simulink model "PTB_BatteryElectricVehicles"  (R2018b)
settings: Solver=ode23tb  StartTime=0.0  StopTime=3158  FixedStep=.001  RelTol=1e-5
model workspace (MAT data in the model file):
  Cd = 0.3
  DrCycles.C505 = [0 1 2 3 4 5 6 7 8 9 10 11 ... (1012 elements, 506x2)]
  DrCycles.FTP = [0 1 2 3 4 5 6 7 8 9 10 11 ... (4956 elements, 2478x2)]
  DrCycles.UDDS = [0 1 2 3 4 5 6 7 8 9 10 11 ... (2746 elements, 1373x2)]
  DrCycles.HWFET = [0 1 2 3 4 5 6 7 8 9 10 11 ... (1532 elements, 766x2)]
  DrCycles.US06 = [0 1 2 3 4 5 6 7 8 9 10 11 ... (1194 elements, 597x2)]
  DrCycles.US06City = [0 1 2 3 4 5 6 7 8 9 10 11 ... (466 elements, 233x2)]
  DrCycles.US06Hwy = [0 1 2 3 4 5 6 7 8 9 10 11 ... (742 elements, 371x2)]
  DriveCycleTime = 3158
  Drive_Cycle = Simulink.LookupTable
  Drive_Cycle.Table = Simulink.lookuptable.Table
  Drive_Cycle.Table.Value = [0 5 10 10 15 15 15 15 20 20 20 20 ... (3158 elements, 3158x1)]
  Drive_Cycle.Table.Dimensions = [3158 1]
  Drive_Cycle.Table.DataType = 'double'
  Drive_Cycle.Table.FieldName = 'Speed'
  Drive_Cycle.Breakpoints = Simulink.lookuptable.Breakpoint
  Drive_Cycle.Breakpoints.Value = [1 2 3 4 5 6 7 8 9 10 11 12 ... (3158 elements, 1x3158)]
  Drive_Cycle.Breakpoints.TunableSizeName = 'N1'
  Drive_Cycle.Breakpoints.Dimensions = [1 3158]
  Drive_Cycle.Breakpoints.DataType = 'double'
  Drive_Cycle.Breakpoints.FieldName = 'Time'
  Drive_Cycle.SupportTunableSize = 0
  Drive_Cycle.StructTypeInfo = Simulink.lookuptable.StructTypeInfo
  Drive_Cycle.StructTypeInfo.Name = 'Drive_Cycle'
  Drive_Cycle.StructTypeInfo.DataScope = 'Auto'
  I = 1
  Kbr = 5000
  P = 200
  axle_b = 10
  axle_k = 0.3
  bevAxle_wc = 400
  bevNp = 1
  bevNs = 8
  diffRatio = 1
  diffRatio1 = 1
  motorMaxTorqueNm = [0.6; 0.6; 0.8; 0.9; 2.2; 2.9; 5.1; 7.8; 11.3; 15.3; 20; 25; 35.4; 41.2; 47.2; 53.4; 66.2; 71.6; 77.2; 82.2; 87.8; 93.1; 98.3; 104; 109.4; 114.6; 120.1; 125.4; 131.1; 137.1; 144.2; 150.1; 155.4; 162.5; 168.1; 173.4; 178.2; 184.5; 190.6; 190.6]
  motorSpeedRadPs = [90.118; 90.118; 90.118; 90.118; 90.01333333; 89.804; 89.49; 89.07133333; 88.65266667; 88.12933333; 87.39666667; 86.87333333; 86.24533333; 85.722; 85.094; 84.25666667; 63.21866667; 57.462; 53.17066667; 49.612; 45.63466667; 41.97133333; 38.72666667; 35.90066667; 33.284; 30.772; 28.36466667; 26.062; 23.96866667; 21.77066667; 19.25866667; 17.47933333; 15.59533333; 13.816; 11.932; 10.25733333; 8.478; 6.594; 4.396]
  vehicleMass = 365
  wheelRadius = 0.3
undefined symbols (not defined in the file): Driver, Wheels_Driver_VehDyn_Lib
libraries: autolibshared x3, simulink x2, autolibdatasheetbattery x1, autolibmappedmotor x1
(part 1 of 3)
settings Model: PauseTimes=2  ParameterArgumentNames=motorMaxTorqueNm  OrderedModelArguments=off  Creator=ogden.michael  LastModifiedBy=ahmed
settings SolverCC: AlgebraicLoopSolver=LineSearch
settings DebuggingCC: AlgebraicLoopMsg=none  LibraryContextMissingDiagnostic=none
settings SFSimCC: SimUseLocalCustomCode=off
settings RTWCC: RTWUseLocalCustomCode=off
settings CodeAppCC: StateflowObjectComments=on
settings SimscapeCC: SimscapeNormalizeSystem=off

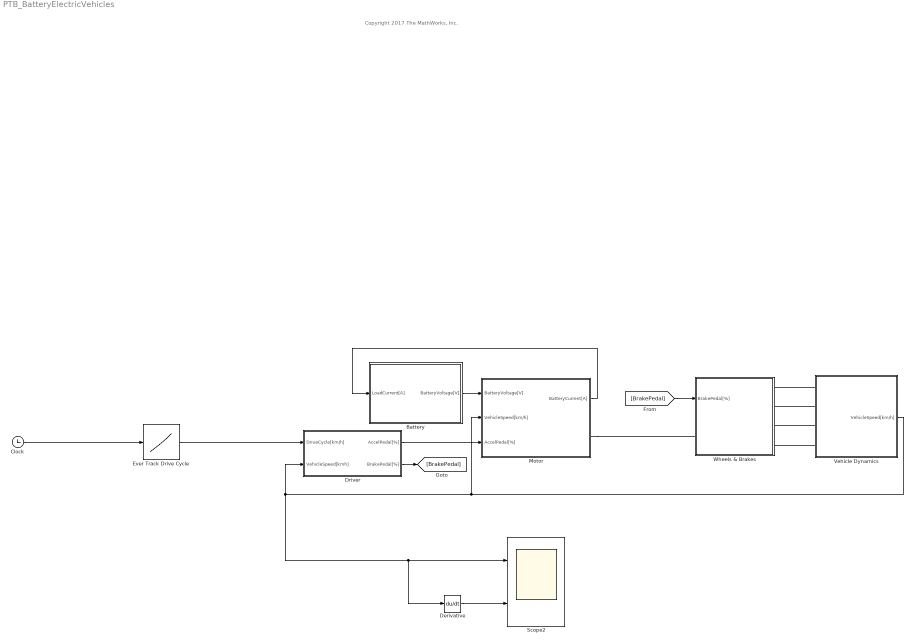
== system PTB_BatteryElectricVehicles ==
  note: Copyright 2017 The MathWorks, Inc.
  Battery : Subsystem
  Clock : Clock
  Derivative : Derivative
  "Driver " : Subsystem  AncestorBlock=Wheels_Driver_VehDyn_Lib/Driver
  Ever Track Drive Cycle : Lookup_n-D  NumberOfTableDimensions=1  DataSpecification=Lookup table object  LookupTableObject=Drive_Cycle  BreakpointsForDimension1=[-5:5]  Table=tanh([-5:5])  InternalRulePriority=Speed  RndMeth=Simplest  InputSameDT=on
  Motor : Subsystem
  Scope2 : Scope  NumInputPorts=2
  Vehicle Dynamics : Subsystem  AncestorBlock=Wheels_Driver_VehDyn_Lib/Vehicle Dynamics
  "Wheels & Brakes " : Subsystem  AncestorBlock=Wheels_Driver_VehDyn_Lib/Wheels & Brakes
  wires:
  [BrakePedal] -> "Wheels & Brakes "/1(BrakePedal[%])
  Battery/1(BatteryVoltage[V]) -> Motor/1(BatteryVoltage[V])
  "Driver "/1(AccelPedal[%]) -> Motor/3(AccelPedal[%])
  "Driver "/2(BrakePedal[%]) -> [BrakePedal]
  Motor/1(BatteryCurrent[A]) -> Battery/1(LoadCurrent[A])
  Clock/1 -> Ever Track Drive Cycle/1
  Vehicle Dynamics/1(VehicleSpeed[km/h]) -> Derivative/1, Scope2/1, "Driver "/2(VehicleSpeed[kmh]), Motor/2(VehicleSpeed[km/h])
  Ever Track Drive Cycle/1 -> "Driver "/1(" DriveCycle[km/h]")
  Derivative/1 -> Scope2/2
  connections:
  Motor/RConn1 -- "Wheels & Brakes "/LConn1
  Vehicle Dynamics/LConn3 -- "Wheels & Brakes "/RConn3
  Vehicle Dynamics/LConn1 -- "Wheels & Brakes "/RConn1
  Vehicle Dynamics/LConn4 -- "Wheels & Brakes "/RConn4
  Vehicle Dynamics/LConn2 -- "Wheels & Brakes "/RConn2

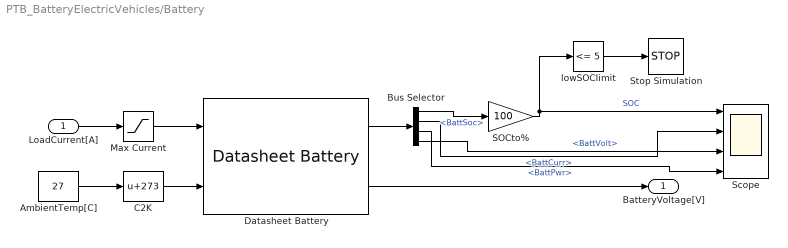
== system PTB_BatteryElectricVehicles/Battery ==
  LoadCurrent[A] : Inport
  AmbientTemp[C] : Constant  Value=27
  Bus Selector : BusSelector  OutputSignals=BattSoc,BattCurr,BattPwr,BattVolt
  C2K : Bias  Bias=273
  Datasheet Battery : autolibdatasheetbattery/Datasheet Battery  CapacityCtrl=Parameter  OutputVlt=Unfiltered  BattChargeMax=80  Em=|  CapLUTBp=|  RInt="[ 0.002789  0.002789;0.002789 0.002789]"  BattTempBp=[300 305]  CapSOCBp=[0 1]  Ns=bevNs  Np=bevNp  BattCapInit=80  Tc=1/1000  Vinit=4.221
      Em=|
      | [5.92
      | 6.22
      | 6.44
      | 6.46
      | 6.54
      | 6.56
      | 6.6
      | 6.6
      | 6.6
      | 6.6
      | 6.6
      | 6.6
      | 6.6
      | 6.6
      | 6.6
      | 6.66
      | 6.66
      | 6.66
      | 6.66
      | 6.7
      | 6.84
      | ]
      CapLUTBp=|
      | [0
      | 0.05
      | 0.1
      | 0.15
      | 0.2
      | 0.25
      | 0.3
      | 0.35
      | 0.4
      | 0.45
      | 0.5
      | 0.55
      | 0.6
      | 0.65
      | 0.7
      | 0.75
      | 0.8
      | 0.85
      | 0.9
      | 0.95
      | 1
      | ]
      settings: SourceProductName=Powertrain Blockset  SourceProductBaseCode=PW
  Max Current : Saturate  UpperLimit=180  LowerLimit=0
  SOCto% : Gain  Gain=100
  Scope : Scope  NumInputPorts=4
  Stop Simulation : Stop
  lowSOClimit : simulink/Logic and Bit Operations/Compare To Constant  relop=<=  const=5  OutDataTypeStr=boolean
  BatteryVoltage[V] : Outport
  wires:
  Datasheet Battery/1 -> Bus Selector/1
  AmbientTemp[C]/1 -> C2K/1
  Datasheet Battery/2 -> BatteryVoltage[V]/1
  C2K/1 -> Datasheet Battery/2
  SOCto%/1 -> lowSOClimit/1, Scope/1  "SOC"
  Bus Selector/1 -> SOCto%/1  "<BattSoc>"
  LoadCurrent[A]/1 -> Max Current/1
  lowSOClimit/1 -> Stop Simulation/1
  Bus Selector/2 -> Scope/2  "<BattCurr>"
  Bus Selector/3 -> Scope/4  "<BattPwr>"
  Bus Selector/4 -> Scope/3  "<BattVolt>"
  Max Current/1 -> Datasheet Battery/1

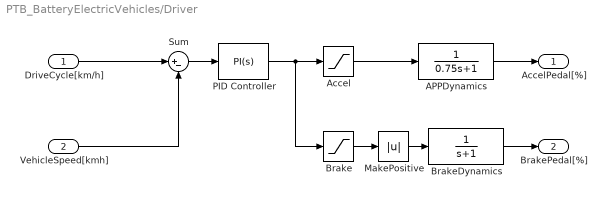
== system PTB_BatteryElectricVehicles/Driver  ==
  " DriveCycle[km/h]" : Inport
  VehicleSpeed[kmh] : Inport  Port=2
  APPDynamics : TransferFcn  Denominator=[0.75 1]
  Accel : Saturate  UpperLimit=100  LowerLimit=0
  Brake : Saturate  UpperLimit=0  LowerLimit=-100
  BrakeDynamics : TransferFcn  Denominator=[1 1]
  MakePositive : Abs
  PID Controller : simulink/Continuous/PID Controller  Controller=PI  Form=Parallel  TimeDomain=Continuous-time  SampleTime=-1  IntegratorMethod=Forward Euler  FilterMethod=Forward Euler  ControllerParametersSource=internal  P=P  I=I  D=0  UseFilter=on  N=100  TunerSelectOption=Transfer Function Based (PID Tuner App)  InitialConditionSource=internal  InitialConditionForIntegrator=0  InitialConditionForFilter=0  DifferentiatorICPrevScaledInput=0  ExternalReset=none  TrackingMode=off  Kt=1  LimitOutput=on  UpperSaturationLimit=100  LowerSaturationLimit=-100  LinearizeAsGain=on  AntiWindupMode=none  Kb=1  POutMin=[]  POutMax=[]  IOutMin=[]  IOutMax=[]  DOutMin=[]  DOutMax=[]  NOutMin=[]  NOutMax=[]  SumOutMin=[]  SumOutMax=[]  SaturationOutMin=[]  SaturationOutMax=[]  PParamMin=[]  PParamMax=[]  IParamMin=[]  IParamMax=[]  DParamMin=[]  DParamMax=[]  NParamMin=[]  NParamMax=[]  KbParamMin=[]  KbParamMax=[]  KtParamMin=[]  KtParamMax=[]  KbOutMin=[]  KbOutMax=[]  KtOutMin=[]  KtOutMax=[]  IntegratorOutMin=[]  IntegratorOutMax=[]  FilterOutMin=[]  FilterOutMax=[]  SumI1OutMin=[]  SumI1OutMax=[]  SumI2OutMin=[]  SumI2OutMax=[]  SumI3OutMin=[]  SumI3OutMax=[]  SumI4OutMin=[]  SumI4OutMax=[]  SumDOutMin=[]  SumDOutMax=[]  DifferentiatorOutMin=[]  DifferentiatorOutMax=[]  FilterDiffOutCoefMin=[]  FilterDiffOutCoefMax=[]  ReciprocalOutMin=[]  ReciprocalOutMax=[]  SumDenOutMin=[]  SumDenOutMax=[]  SumNumOutMin=[]  SumNumOutMax=[]  DivideOutMin=[]  DivideOutMax=[]  IntegratorContinuousStateAttributes=''  IntegratorStateMustResolveToSignalObject=off  IntegratorRTWStateStorageClass=Auto  FilterContinuousStateAttributes=''  FilterStateMustResolveToSignalObject=off  FilterRTWStateStorageClass=Auto  ParallelPVariant=InternalParameters  IdealPVariant=Disabled  IVariant=InternalParameters  DVariant=Disabled  IntegratorVariant=Continuous  SatVariant=Enabled  AWVariant=Passthrough  PCopyVariant=Disabled  TRVariant=Disabled  FdbkBlocksVariant=Forward  IdealPFdbkVariant=Disabled  SatFdbkVariant=Disabled  DerivativeFilterVariant=Disabled  NVariant=Disabled  NCopyVariant=Disabled_SignalSpec  FilterICVariant=Disabled  IntegratorICVariant=InternalICs  ExternalResetVariant=Disabled  TRSumVariant=Passthrough  SumFdbkVariant=Disabled  SumVariant=Sum_PI
  Sum : Sum  Inputs=|+-
  AccelPedal[%] : Outport
  BrakePedal[%] : Outport  Port=2
  wires:
  " DriveCycle[km/h]"/1 -> Sum/1
  VehicleSpeed[kmh]/1 -> Sum/2
  PID Controller/1 -> Accel/1, Brake/1
  Sum/1 -> PID Controller/1
  Brake/1 -> MakePositive/1
  Accel/1 -> APPDynamics/1
  MakePositive/1 -> BrakeDynamics/1
  APPDynamics/1 -> AccelPedal[%]/1
  BrakeDynamics/1 -> BrakePedal[%]/1

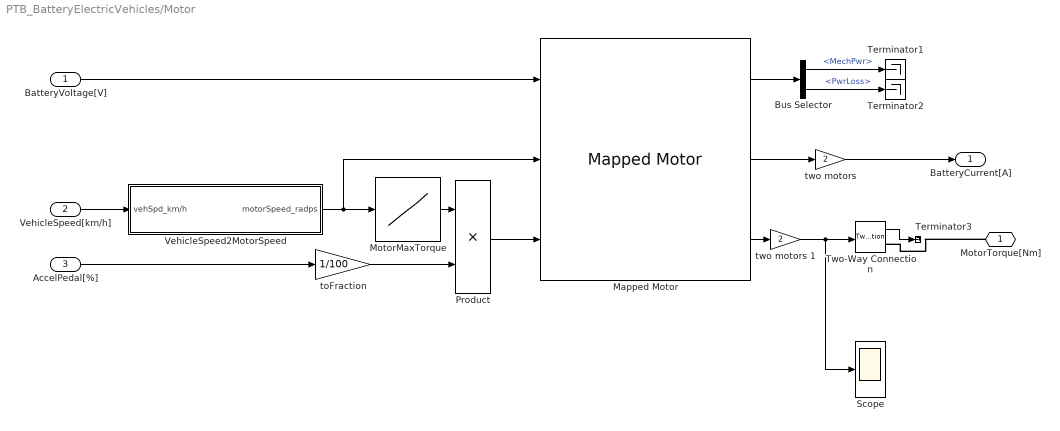
== system PTB_BatteryElectricVehicles/Motor ==
  BatteryVoltage[V] : Inport
  VehicleSpeed[km/h] : Inport  Port=2
  AccelPedal[%] : Inport  Port=3
  Bus Selector : BusSelector  OutputSignals=MechPwr,PwrLoss
  Mapped Motor : autolibmappedmotor/Mapped Motor  port_config=Speed  param_by=Maximum torque and power  w_t=|  T_t=|  torque_max=175  power_max=4600  Tc=0.01  param_loss=Tabulated efficiency data  eff=62.9  w_eff=85.5  T_eff=5  Piron=0  Pbase=0  w_eff_bp=|  T_eff_bp=[10 20 30 40 50 60 70 80 90 100 110 120 130 140 150 160 170 180]  losses_table=[1.49 1.67 2.21 3.10; 0.42 0.69 1.14 2.03; 0.06 0.24 0.78 1.68; 0.42 0.69 1.14 2.03; 1.49 1.67 2.21 3.10]  efficiency_table=|  J=5e-6  b=1e-5  omega_o=0  T_t_extended=[6 5 5 5 5 5 5 6]  w_t_extended=[-62 -10 -5 -1 1 5 10 62]  KLossIron=0  KLossCopper=10.086  x_w_eff_vec=[-88.96666667 -83.73333333 -78.5 -73.26666667 -68.03333333 -62.8 -57.56666667 -52.33333333 -47.1 -41.86666667 -36.63333333 -31.4 -26.16666667 -20.93333333 -15.7 -10.46666667 -5.233333333 5.233333333 10.46666667 15.7 20.93333333 26.16666667 31.4 36.63333333 41.86666667 47.1 52.33333333 57.56666667 62.8 68.03333333 73.26666667 78.5 83.73333333 88.96666667]  x_T_eff_vec=[-180 -170 -160 -150 -140 -130 -120 -110 -100 -90 -80 -70 -60 -50 -40 -30 -20 -10 10 20 30 40 50 60 70 80 90 100 110 120 130 140 150 160 170 180]  x_losses_mat=[1585386.0000594 1497309.0000561 1409232.0000528 1321155.0000495 1233078.0000462 1145001.0000429 1056924.0000396 968847.0000363 880770.000033 792693.0000297 704616.0000264 616539.0000231 528462.0000198 440385.0000165 889.6666667 667.250000025 444.83333335 593.111111133333 355.86666668 355.86666668 533.80000002 711.73333336 4403.850000165 5284.620000198 6165.390000231 7046.160000264 7926.930000297 8807.70000033 9688.470000363 10569.240000396 11450.010000429 12330.780000462 13211.550000495 14092.320000528 14973.090000561 15853.860000594;1492127.9999406 1409231.9999439 1326335.9999472 1243439.9999505 1160543.9999538 1077647.9999571 994751.9999604 911855.9999637 828959.999967 746063.9999703 663167.9999736 580271.9999769 497375.9999802 1046.666666625 837.3333333 627.999999975 1116.4444444 3349.3333332 669.86666664 669.86666664 502.39999998 669.86666664 837.3333333 4973.759999802 5802.719999769 6631.679999736 7460.639999703 8289.59999967 9118.559999637 9947.519999604 10776.479999571 11605.439999538 12434.399999505 13263.359999472 14092.319999439 14921.279999406;1398870 1321155 1243440 1165725 1088010 1010295 932580 854865 777150 699435 621720 544005 1177.5 981.25 785 2355 3663.33333333333 3140 628 1099 1177.5 628 785 942 5440.05 6217.2 6994.35 7771.5 8548.65 9325.8 10102.95 10880.1 11657.25 12434.4 13211.55 13988.7;1305612.0000594 1233078.0000561 1160544.0000528 1088010.0000495 1015476.0000462 942942.0000429 870408.0000396 797874.0000363 725340.000033 652806.0000297 580272.0000264 1282.166666725 1099.00000005 915.833333375 2930.6666668 5128.6666669 3419.11111126667 2930.6666668 586.13333336 1025.73333338 1538.60000007 1465.3333334 732.6666667 879.20000004 1025.73333338 5802.720000264 6528.060000297 7253.40000033 7978.740000363 8704.080000396 9429.420000429 10154.760000462 10880.100000495 11605.440000528 12330.780000561 13056.120000594;1212353.9999406 1145000.9999439 1077647.9999472 1010294.9999505 942941.9999538 875588.9999571 808235.9999604 740882.9999637 673529.999967 606176.9999703 2332.57142845714 1190.583333275 1020.49999995 2267.77777766667 4081.9999998 4762.3333331 3174.88888873333 2721.3333332 544.26666664 952.46666662 1428.69999993 1632.79999992 1360.6666666 816.39999996 952.46666662 1632.79999992 6061.769999703 6735.29999967 7408.829999637 8082.359999604 8755.889999571 9429.419999538 10102.949999505 10776.479999472 11450.009999439 12123.539999406;1119096 1056924 994752 932580 870408 808236 746064 683892 621720 2422.28571428571 2153.14285714286 1099 1614.85714285714 3140 3768 4396 2930.66666666667 2512 502.4 879.2 1318.8 1507.2 1570 1130.4 879.2 1507.2 1695.6 6217.2 6838.92 7460.64 8082.36 8704.08 9325.8 9947.52 10569.24 11190.96;1025838.0000594 968847.0000561 911856.0000528 854865.0000495 797874.0000462 740883.0000429 683892.0000396 626901.0000363 569910.000033 2220.42857155714 1151.3333334 1007.416666725 3454.0000002 2878.3333335 3454.0000002 4029.6666669 2686.4444446 2302.6666668 460.53333336 805.93333338 1208.90000007 1381.60000008 1439.16666675 1727.0000001 805.93333338 921.06666672 1554.30000009 5699.10000033 6269.010000363 6838.920000396 7408.830000429 7978.740000462 8548.650000495 9118.560000528 9688.470000561 10258.380000594;932579.9999406 880769.9999439 828959.9999472 777149.9999505 725339.9999538 673529.9999571 621719.9999604 569909.9999637 3488.88888866667 2018.57142844286 1046.6666666 2442.22222206667 2093.3333332 2616.6666665 2093.3333332 2354.99999985 2442.22222206667 2093.3333332 418.66666664 732.66666662 941.99999994 1046.6666666 1308.33333325 1255.99999992 1465.33333324 837.33333328 1412.99999991 2093.3333332 5699.099999637 6217.199999604 6735.299999571 7253.399999538 7771.499999505 8289.599999472 8807.699999439 9325.799999406;839322 792693 746064 699435 652806 606177 559548 3454 2018.57142857143 1059.75 1614.85714285714 2198 1884 1570 1884 2119.5 2198 1884 376.8 659.4 847.8 942 942 1130.4 1318.8 1130.4 847.8 1413 2072.4 5595.48 6061.77 6528.06 6994.35 7460.64 7926.93 8393.22;746064.0000594 704616.0000561 ...(+10945 chars)]  aMode=aMode
      w_t=|
      | [0
      | 4.396
      | 6.594
      | 8.478
      | 10.25733333
      | 11.932
      | 13.816
      | 15.59533333
      | 17.47933333
      | 19.25866667
      | 21.77066667
      | 23.96866667
      | 26.062
      | 28.36466667
      | 30.772
      | 33.284
      | 35.90066667
      | 38.72666667
      | 41.97133333
      | 45.63466667
      | 49.612
      | 53.17066667
      | 57.462
      | 63.21866667
      | 84.25666667
      | 85.094
      | 85.722
      | 86.24533333
      | 86.87333333
      | 87.39666667
      | 88.12933333
      | 88.65266667
      | 89.07133333
      | 89.49
      | 89.804
      | ]
      T_t=|
      | [190.6
      | 190.6
      | 184.5
      | 178.2
      | 173.4
      | 168.1
      | 162.5
      | 155.4
      | 150.1
      | 144.2
      | 137.1
      | 131.1
      | 125.4
      | 120.1
      | 114.6
      | 109.4
      | 104.0
      | 98.3
      | 93.1
      | 87.8
      | 82.2
      | 77.2
      | 71.6
      | 66.2
      | 53.4
      | 47.2
      | 41.2
      | 35.4
      | 25.0
      | 20.0
      | 15.3
      | 11.3
      | 7.8
      | 5.1
      | 2.9
      | ]
      w_eff_bp=|
      | [5.233333333	10.46666667	15.7	20.93333333	26.16666667	31.4	36.63333333	41.86666667	47.1	52.33333333	57.56666667	62.8	68.03333333	73.26666667	78.5	83.73333333	88.96666667
      | ]
      efficiency_table=|
      | [20 20 20 20 20 20 20 20 20 20 20 20 20 20 20 20 20 20;
      |     20 30 30 30 30 30 30 30 30 30 30 30 30 30 30 30 30 20;
      |     20 30 30 40 40 40 40 40 40 40 40 40 40  50 50 40 30 1;
      |     20 30 30 40 50 50 50 50 50 50 50 60 60 60 50 40 1 1;
      |     20 30 40 40 50 60 60 60 60 60 70 60 60 50 40 1 1 1;
      |     20 30 40 40 50 60 60 60 70 70 70 60 50 50 1 1 1 1;
      |     20 30 40 40 50 60 60 70 70 70 70 60 50 1 1 1 1 1;
      |     20 30 40 40 50 60 60 70 80 70 60 60 1 1 1 1 1 1;
      |     20 30 40 50 60 60 60 70 80 70 60 1 1 1 1 1 1 1;
      |     20 30 40 50 50 60 60 80 70 60 1 1 1 1 1 1 1 1;
      |     20 30 30 40 50 50 80 80 70 1 1 1 1 1 1 1 1 1;
      |     20 30 30 40 50 70 80 70 70 1 1 1 1 1 1 1 1 1;
      |     20 30 30 40 60 80 80 70 1 1 1 1 1 1 1 1 1 1;
      |     20 30 30 50 80 80 80 1 1 1 1 1 1 1 1 1 1 1;
      |     20 30 50 80 80 80 1 1 1 1 1 1 1 1 1 1 1 1;
      |     20 60 80 80 80 1 1 1 1 1 1 1 1 1 1 1 1 1;
      |     60 80 80 80 1 1 1 1 1 1 1 1 1 1 1 1 1 1]
      settings: SourceProductName=Powertrain Blockset  SourceProductBaseCode=PW
  MotorMaxTorque : Lookup_n-D  NumberOfTableDimensions=1  BreakpointsForDimension1=|  Table=|  ExtrapMethod=Clip  InternalRulePriority=Speed  RndMeth=Simplest  InputSameDT=on
      BreakpointsForDimension1=|
      | [4.396
      | 6.594
      | 8.478
      | 10.25733333
      | 11.932
      | 13.816
      | 15.59533333
      | 17.47933333
      | 19.25866667
      | 21.77066667
      | 23.96866667
      | 26.062
      | 28.36466667
      | 30.772
      | 33.284
      | 35.90066667
      | 38.72666667
      | 41.97133333
      | 45.63466667
      | 49.612
      | 53.17066667
      | 57.462
      | 63.21866667
      | 84.25666667
      | 85.094
      | 85.722
      | 86.24533333
      | 86.87333333
      | 87.39666667
      | 88.12933333
      | 88.65266667
      | 89.07133333
      | 89.49
      | 89.804
      | 90.01333333
      | 90.118
      | 
      | ]
      Table=|
      | [190.6
      | 184.5
      | 178.2
      | 173.4
      | 168.1
      | 162.5
      | 155.4
      | 150.1
      | 144.2
      | 137.1
      | 131.1
      | 125.4
      | 120.1
      | 114.6
      | 109.4
      | 104.0
      | 98.3
      | 93.1
      | 87.8
      | 82.2
      | 77.2
      | 71.6
      | 66.2
      | 53.4
      | 47.2
      | 41.2
      | 35.4
      | 25.0
      | 20.0
      | 15.3
      | 11.3
      | 7.8
      | 5.1
      | 2.9
      | 2.2
      | 0.9
      | 
      | ]
  Product : Product
  Scope : Scope
  Terminator1 : Terminator
  Terminator2 : Terminator
  Terminator3 : Terminator
  Two-Way Connectio n : TwoWayConnection
  VehicleSpeed2MotorSpeed : Subsystem
  toFraction : Gain  Gain=1/100
  "two motors " : Gain  Gain=2
  two motors 1 : Gain  Gain=2
  MotorTorque[Nm] : PMIOPort  Side=Right
  BatteryCurrent[A] : Outport
  wires:
  BatteryVoltage[V]/1 -> Mapped Motor/1
  Mapped Motor/2 -> "two motors "/1
  VehicleSpeed[km/h]/1 -> VehicleSpeed2MotorSpeed/1(vehSpd_km/h)
  VehicleSpeed2MotorSpeed/1(motorSpeed_radps) -> MotorMaxTorque/1, Mapped Motor/2
  Mapped Motor/1 -> Bus Selector/1
  Two-Way Connectio n/1 -> Terminator3/1
  Product/1 -> Mapped Motor/3
  MotorMaxTorque/1 -> Product/1
  AccelPedal[%]/1 -> toFraction/1
  toFraction/1 -> Product/2
  Bus Selector/2 -> Terminator2/1  "<PwrLoss>"
  Bus Selector/1 -> Terminator1/1  "<MechPwr>"
  Mapped Motor/3 -> two motors 1/1
  "two motors "/1 -> BatteryCurrent[A]/1
  two motors 1/1 -> Scope/1, Two-Way Connectio n/1
  connections:
  MotorTorque[Nm]/RConn1 -- Two-Way Connectio n/RConn1

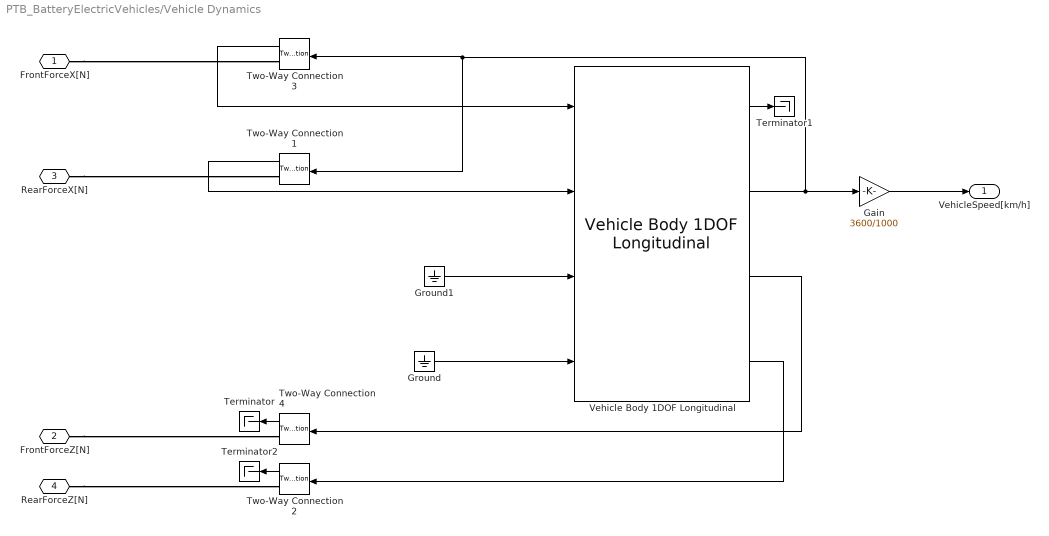
== system PTB_BatteryElectricVehicles/Vehicle Dynamics ==
  Gain : Gain  Gain=3600/1000
  Ground : Ground
  Ground1 : Ground
  Terminator : Terminator
  Terminator1 : Terminator
  Terminator2 : Terminator
  Two-Way Connection{1..4} (4 alike) : TwoWayConnection
  Vehicle Body 1DOF Longitudinal : autolibshared/Vehicle Body 1DOF Longitudinal  VariantControl=SL  aMode=aMode  NF=2  NR=2  m=vehicleMass  a=1.3  b=1  h=.35  Cd=.3  Af=1.2  x_o=0  xdot_o=0  Pabs=101325  T=273  g=9.81
      settings: SourceProductName=Powertrain Blockset  SourceProductBaseCode=PW
  FrontForceX[N] : PMIOPort  Side=Left
  FrontForceZ[N] : PMIOPort  Port=2  Side=Left
  RearForceX[N] : PMIOPort  Port=3  Side=Left
  RearForceZ[N] : PMIOPort  Port=4  Side=Left
  VehicleSpeed[km/h] : Outport
  wires:
  Ground1/1 -> Vehicle Body 1DOF Longitudinal/3
  Ground/1 -> Vehicle Body 1DOF Longitudinal/4
  Vehicle Body 1DOF Longitudinal/2 -> Gain/1, Two-Way Connection1/1, Two-Way Connection3/1
  Vehicle Body 1DOF Longitudinal/1 -> Terminator1/1
  Vehicle Body 1DOF Longitudinal/3 -> Two-Way Connection4/1
  Vehicle Body 1DOF Longitudinal/4 -> Two-Way Connection2/1
  Two-Way Connection3/1 -> Vehicle Body 1DOF Longitudinal/1
  Two-Way Connection1/1 -> Vehicle Body 1DOF Longitudinal/2
  Two-Way Connection4/1 -> Terminator/1
  Two-Way Connection2/1 -> Terminator2/1
  Gain/1 -> VehicleSpeed[km/h]/1
  connections:
  FrontForceX[N]/RConn1 -- Two-Way Connection3/RConn1
  FrontForceZ[N]/RConn1 -- Two-Way Connection4/RConn1
  RearForceX[N]/RConn1 -- Two-Way Connection1/RConn1
  RearForceZ[N]/RConn1 -- Two-Way Connection2/RConn1
